simulink model "Synchrouns_Buck_Converter"  (R2022b)
settings: Solver=FixedStepAuto  StartTime=0.0  StopTime=inf  MaxStep=1e-5  RelTol=1e-3  EnableMultiTasking=on
libraries: spsSeriesRLCBranchLib x3, arduinolib x2, spsCurrentMeasurementLib x2, spsMosfetLib x2, spsVoltageMeasurementLib x2, spsDCVoltageSourceLib x1, spsFirstOrderFilterLib x1, dspstat3 x1, slpidlib x1, simulink x1, spspowerguiLib x1
settings Model: ExtModeTrigDuration=2  Creator=es-ahmedabdellatif20  LastModifiedBy=es-ahmedabdellatif20
settings OptimizationCC: EnhancedBackFolding=on  PassReuseOutputArgsAs=Individual arguments  ZeroExternalMemoryAtStartup=off  ZeroInternalMemoryAtStartup=off  MaxStackSize=64  OptimizeBlockOrder=speed  DifferentSizesBufferReuse=on  OptimizationCustomize=off  EfficientTunableParamExpr=on
settings DebuggingCC: ParameterTunabilityLossMsg=error
settings HardwareCC: ProdBitPerInt=16  ProdBitPerPointer=16  ProdBitPerSizeT=16  ProdBitPerPtrDiffT=16  ProdLargestAtomicFloat=None  ProdWordSize=8  ProdHWDeviceType=Atmel->AVR
settings SFSimCC: MATLABDynamicMemAlloc=off
settings RTWCC: Description=Embedded Coder  SystemTargetFile=ert.tlc  HardwareBoard=Arduino Uno  TLCOptions=-aInlineSetEventsForThisBaseRateFcn=TLC_FALSE -aSuppressMultiTaskScheduler=TLC_FALSE -aRateBasedStepFcn=1  TemplateMakefile=ert_default_tmf  Toolchain=Arduino AVR  BuildConfiguration=Faster Runs
settings CodeAppCC: ForceParamTrailComments=on  IgnoreCustomStorageClasses=off  OperatorAnnotations=on  SimulinkDataObjDesc=on  SFDataObjDesc=on  InsertBlockDesc=on
settings ERTTargetCC: SupportContinuousTime=on  SupportVariableSizeSignals=on  ExtModeTransport=3  ExtModeStaticAlloc=on  ExtModeAutomaticAllocSize=off  ExtModeStaticAllocSize=250  ExtModeMexFile=ext_xcp  ExtModeIntrfLevel=Level2 - Open

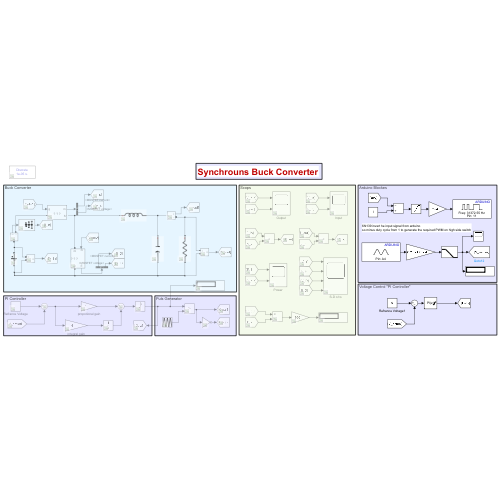
[thumbnail: Simulink's stored preview of the top-level diagram]
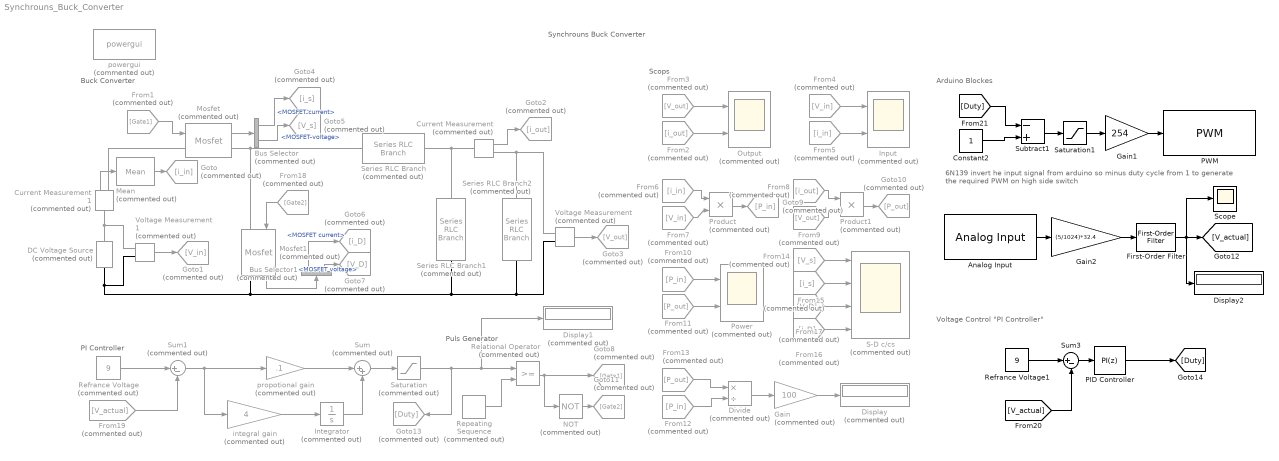
== system Synchrouns_Buck_Converter ==
  note: Voltage Control "PI Controller"
  note: 6N139 invert he input signal from arduino
      | so minus duty cycle from 1 to generate the required PWM on high side switch
  note: Arduino Blockes
  note: Scops
  note: Synchrouns Buck Converter
  note: Puls Generator
  note: PI Controller
  note: Buck Converter
  Analog Input : arduinolib/Analog Input  pinNumber=4  ReadResultsOnly=off  ConversionTriggerSource=Software  ExternalTriggerType=uint32( 0 )  OutputDataType=uint16  EnableConversionCompleteNotify=off  EnableOuputStatus=off  SampleTime=1e-3  blockPlatform=arduino
  Bus Selector : BusSelector  Commented=on  OutputSignals=MOSFET current,MOSFET voltage
  Bus Selector1 : BusSelector  Commented=on  OutputSignals=MOSFET current,MOSFET voltage
  Constant2 : Constant
  Current Measurement : spsCurrentMeasurementLib/Current Measurement  Commented=on  PhasorSimulation=off  OutputType=Complex  PSBequivalent=0
  Current Measurement1 : spsCurrentMeasurementLib/Current Measurement  Commented=on  PhasorSimulation=off  OutputType=Complex  PSBequivalent=0
  DC Voltage Source : spsDCVoltageSourceLib/DC Voltage Source  Commented=on  Amplitude=12  Measurements=Voltage
  Display : Display  Commented=on
  Display1 : Display  Commented=on
  Display2 : Display
  Divide : Product  Commented=on  Inputs=*/
  First-Order Filter : spsFirstOrderFilterLib/First-Order Filter  FilterType=Lowpass  Tc=1/250  Ts=1e-3  Initialize=off  Vac_Init=[0, 0, 60]  Vdc_Init=0  PlotResponse=off  FreqRange="[0,  200,  1]"
  From1 : From  Commented=on  GotoTag=Gate1
  From10 : From  Commented=on  GotoTag=P_in
  From11 : From  Commented=on  GotoTag=P_out
  From12 : From  Commented=on  GotoTag=P_in
  From13 : From  Commented=on  GotoTag=P_out
  From14 : From  Commented=on  GotoTag=V_s
  From15 : From  Commented=on  GotoTag=i_s
  From16 : From  Commented=on  GotoTag=i_D
  From17 : From  Commented=on  GotoTag=V_D
  From18 : From  Commented=on  GotoTag=Gate2
  From19 : From  Commented=on  GotoTag=V_actual
  From2 : From  Commented=on  GotoTag=i_out
  From3 : From  Commented=on  GotoTag=V_out
  From4 : From  Commented=on  GotoTag=V_in
  From5 : From  Commented=on  GotoTag=i_in
  From6 : From  Commented=on  GotoTag=i_in
  From7 : From  Commented=on  GotoTag=V_in
  From8 : From  Commented=on  GotoTag=i_out
  From9 : From  Commented=on  GotoTag=V_out
  Gain : Gain  Commented=on  Gain=100
  Gain1 : Gain  Gain=254
  Gain2 : Gain  Gain=(5/1024)*32.4
  Goto : Goto  Commented=on  GotoTag=i_in
  Goto1 : Goto  Commented=on  GotoTag=V_in
  Goto10 : Goto  Commented=on  GotoTag=P_out
  Goto11 : Goto  Commented=on  GotoTag=Gate2
  Goto13 : Goto  Commented=on  GotoTag=Duty
  Goto2 : Goto  Commented=on  GotoTag=i_out
  Goto3 : Goto  Commented=on  GotoTag=V_out
  Goto4 : Goto  Commented=on  GotoTag=i_s
  Goto5 : Goto  Commented=on  GotoTag=V_s
  Goto6 : Goto  Commented=on  GotoTag=i_D
  Goto7 : Goto  Commented=on  GotoTag=V_D
  Goto8 : Goto  Commented=on  GotoTag=Gate1
  Goto9 : Goto  Commented=on  GotoTag=P_in
  Input : Scope  Commented=on  NumInputPorts=2
  Integrator : Integrator  Commented=on
  Mean : dspstat3/Mean  Commented=on  run=on  InputProcessing=Columns as channels (frame based)  reset_popup=None  directionMode=Each column  dimension=1  roiEnable=off  roiType=Rectangles  roiPortion=Entire ROI  roiOutput=Individual statistics for each ROI  roiFlag=off  roundingMode=Floor  overflowMode=off  outputDataTypeStr=Inherit: Same as accumulator  outputMin=[]  outputMax=[]  outputLastDataTypeStr=Inherit: Same as accumulator
  Mosfet : spsMosfetLib/Mosfet  Commented=on  Ron=0.1  Lon=0  Rd=0.01  Vfd=0  IC=0  Rs=1e5  Cs=inf  Measurements=on
  Mosfet1 : spsMosfetLib/Mosfet  Commented=on  Ron=0.1  Lon=0  Rd=0.01  Vfd=0  IC=0  Rs=1e5  Cs=inf  Measurements=on
  NOT : Logic  Commented=on  Operator=NOT  IconShape=distinctive  AllPortsSameDT=off  OutDataTypeStr=boolean
  Output : Scope  Commented=on  NumInputPorts=2
  PID Controller : slpidlib/PID Controller  Controller=PI  Form=Parallel  TimeDomain=Discrete-time  UseExternalTs=off  SampleTime=1e-3  IntegratorMethod=Forward Euler  FilterMethod=Forward Euler  ControllerParametersSource=internal  P=.1  I=6  UseKiTs=off  D=0  N=100  UseFilter=on  TunerSelectOption=Transfer Function Based (PID Tuner App)  InitialConditionSource=internal  InitialConditionForIntegrator=0  InitialConditionForFilter=0  DifferentiatorICPrevScaledInput=0  ExternalReset=none  TrackingMode=off  Kt=1  LimitOutput=on  SatLimitsSource=internal  UpperSaturationLimit=1  LowerSaturationLimit=0  LinearizeAsGain=on  AntiWindupMode=clamping  Kb=1  LimitIntegrator=off  UpperIntegratorSaturationLimit=inf  LowerIntegratorSaturationLimit=-inf  POutMin=[]  POutMax=[]  IOutMin=[]  IOutMax=[]  DOutMin=[]  DOutMax=[]  NOutMin=[]  NOutMax=[]  SumOutMin=[]  SumOutMax=[]  SaturationOutMin=[]  SaturationOutMax=[]  PParamMin=[]  PParamMax=[]  IParamMin=[]  IParamMax=[]  DParamMin=[]  DParamMax=[]  NParamMin=[]  NParamMax=[]  KbParamMin=[]  KbParamMax=[]  KtParamMin=[]  KtParamMax=[]  KbOutMin=[]  KbOutMax=[]  KtOutMin=[]  KtOutMax=[]  IntegratorOutMin=[]  IntegratorOutMax=[]  FilterOutMin=[]  FilterOutMax=[]  SumI1OutMin=[]  SumI1OutMax=[]  SumI2OutMin=[]  SumI2OutMax=[]  SumI3OutMin=[]  SumI3OutMax=[]  SumI4OutMin=[]  SumI4OutMax=[]  SumDOutMin=[]  SumDOutMax=[]  DifferentiatorOutMin=[]  DifferentiatorOutMax=[]  FilterDiffOutCoefMin=[]  FilterDiffOutCoefMax=[]  ReciprocalOutMin=[]  ReciprocalOutMax=[]  SumDenOutMin=[]  SumDenOutMax=[]  SumNumOutMin=[]  SumNumOutMax=[]  DivideOutMin=[]  DivideOutMax=[]  UdiffTsProdOutMin=[]  UdiffTsProdOutMax=[]  NTsProdOutMin=[]  NTsProdOutMax=[]  UintegralTsProdOutMin=[]  UintegralTsProdOutMax=[]  UngainTsProdOutMin=[]  UngainTsProdOutMax=[]  ClampingZeroOutDataTypeStr=Inherit: Inherit via back propagation  ClampingZeroOutMin=[]  ClampingZeroOutMax=[]  FilterDenConstantOutDataTypeStr=Inherit: Inherit via back propagation  FilterDenConstantOutMin=[]  FilterDenConstantOutMax=[]  PCopyOutDataTypeStr=Inherit: Inherit via back propagation  PCopyOutMin=[]  PCopyOutMax=[]  NCopyOutDataTypeStr=Inherit: Inherit via back propagation  NCopyOutMin=[]  NCopyOutMax=[]  IntegratorContinuousStateAttributes=''  IntegratorStateMustResolveToSignalObject=off  IntegratorRTWStateStorageClass=Auto  FilterContinuousStateAttributes=''  FilterStateMustResolveToSignalObject=off  FilterRTWStateStorageClass=Auto  ParallelPVariant=InternalParameters  IdealPVariant=Disabled  IVariant=InternalParameters  DVariant=Disabled  IntegratorVariant=Discrete  SatVariant=Enabled  AWVariant=DiscClampingParallel  PCopyVariant=Disabled  TRVariant=Disabled  FdbkBlocksVariant=Forward  IdealPFdbkVariant=Disabled  SatFdbkVariant=Disabled  DerivativeFilterVariant=Disabled  NVariant=Disabled  NCopyVariant=Disabled_SignalSpec  FilterICVariant=Disabled  IntegratorICVariant=InternalICs  ExternalResetVariant=Disabled  TRSumVariant=Passthrough  SumFdbkVariant=Disabled  SumVariant=Sum_PI  TsampFilterVariant=InternalTs  TsampNgainVariant=Passthrough  TsampIntegralVariant=Passthrough  ExternalSaturationOutDataTypeStr=Inherit: Same as second input
  PWM : arduinolib/PWM  pinNumber=11  frequencyType=Specify  desiredFrequency=31372.55  achievableFrequency=31372.55
  Power : Scope  Commented=on  NumInputPorts=2
  Product : Product  Commented=on
  Product1 : Product  Commented=on
  Refrance Voltage : Constant  Commented=on  Value=9
  Refrance Voltage1 : Constant  Value=9
  Relational Operator : RelationalOperator  Commented=on  OutDataTypeStr=boolean  RndMeth=Simplest  InputSameDT=off
  Repeating Sequence : simulink/Sources/Repeating Sequence  Commented=on  rep_seq_t=[0 1/(31372.55*2) 1/31372.55]  rep_seq_y=[0 1 0]
  S-D c/cs : Scope  Commented=on  NumInputPorts=4
  Saturation : Saturate  Commented=on  UpperLimit=1  LowerLimit=0
  Saturation1 : Saturate  UpperLimit=1  LowerLimit=0
  Scope : Scope
  Series RLC Branch : spsSeriesRLCBranchLib/Series RLC Branch  Commented=on  LConnTagsString=__new0  RConnTagsString=__new0  BranchType=L  Resistance=1  Inductance=4e-3  SetiL0=off  InitialCurrent=0  Capacitance=1e-6  Setx0=off  InitialVoltage=0  Measurements=None
  Series RLC Branch1 : spsSeriesRLCBranchLib/Series RLC Branch  Commented=on  LConnTagsString=__new0  RConnTagsString=__new0  BranchType=C  Resistance=1  Inductance=1e-3  SetiL0=off  InitialCurrent=0  Capacitance=2200e-6  Setx0=off  InitialVoltage=0  Measurements=None
  Series RLC Branch2 : spsSeriesRLCBranchLib/Series RLC Branch  Commented=on  LConnTagsString=__new0  RConnTagsString=__new0  BranchType=R  Resistance=1  Inductance=1e-3  SetiL0=off  InitialCurrent=0  Capacitance=1e-6  Setx0=off  InitialVoltage=0  Measurements=None
  Subtract1 : Sum  Inputs=-+
  Sum : Sum  Commented=on  Inputs=|++
  Sum1 : Sum  Commented=on  Inputs=|+-
  Sum3 : Sum  Inputs=|+-
  Voltage Measurement : spsVoltageMeasurementLib/Voltage Measurement  Commented=on  PhasorSimulation=off  OutputType=Complex  PSBequivalent=0
  Voltage Measurement1 : spsVoltageMeasurementLib/Voltage Measurement  Commented=on  PhasorSimulation=off  OutputType=Complex  PSBequivalent=0
  integral gain : Gain  Commented=on  Gain=4
  powergui : spspowerguiLib/powergui  Priority=1  Commented=on  SimulationMode=Discrete  SampleTime=1e-5  frequency=60  Iterations=50  frequencyindice=0  Pbase=100e6  ErrMax=1e-4  UnitsV=kV  UnitsW=MW  buscounter=0  FunctionMessages=off  echomessages=off  EnableUseOfTLC=off  CurrentSourceSwitches=off  DisableSnubberDevices=off  DisableRonSwitches=off  DisableVfSwitches=off  DisplayEquations=off  AutomaticDiscreteSolvers=off  SolverType=Tustin/Backward Euler (TBE)  Interpol=off  ExternalGateDelay=off  methode=off  Ts=100  x0status=blocks  SPID=on  SwTol=0  HookPort=off  NonlinearTolerance=1e-4  nMaxIteration=100  ContinueOnMaxIteration=off  RestoreLinks=warning  ResistiveCurrentMeasurement=off  Frange=[0:2:500]  Ylog=off  Xlog=on  ShowGrid=off  save=off  variable=ZData  structure=0  ZoomFFT=off  StartTime=0.0  cycles=1  DisplayStyle=1  fundamental=60  FreqAxis=off  MaxFrequency=1000  frequencyindicesteady=1  RmsSteady=1  display=off
  propotional gain : Gain  Commented=on  Gain=.1
  wires:
  Voltage Measurement1/1 -> Goto1/1
  Current Measurement/1 -> Goto2/1
  Voltage Measurement/1 -> Goto3/1
  Mosfet/1 -> Bus Selector/1
  Mosfet1/1 -> Bus Selector1/1
  Bus Selector/1 -> Goto4/1  "<MOSFET current>"
  Bus Selector/2 -> Goto5/1  "<MOSFET voltage>"
  Bus Selector1/1 -> Goto6/1  "<MOSFET current>"
  integral gain/1 -> Integrator/1
  Integrator/1 -> Sum/2
  propotional gain/1 -> Sum/1
  Sum/1 -> Saturation/1
  Relational Operator/1 -> Goto8/1, NOT/1
  Refrance Voltage/1 -> Sum1/1
  Sum1/1 -> integral gain/1, propotional gain/1
  From1/1 -> Mosfet/1
  Bus Selector1/2 -> Goto7/1  "<MOSFET voltage>"
  Repeating Sequence/1 -> Relational Operator/2
  From3/1 -> Output/1
  From2/1 -> Output/2
  From5/1 -> Input/2
  From4/1 -> Input/1
  From6/1 -> Product/1
  From7/1 -> Product/2
  From9/1 -> Product1/2
  From8/1 -> Product1/1
  Product/1 -> Goto9/1
  Product1/1 -> Goto10/1
  From10/1 -> Power/1
  From11/1 -> Power/2
  From13/1 -> Divide/1
  From12/1 -> Divide/2
  Divide/1 -> Gain/1
  Gain/1 -> Display/1
  From14/1 -> S-D c/cs/1
  From15/1 -> S-D c/cs/2
  From17/1 -> S-D c/cs/3
  From16/1 -> S-D c/cs/4
  Current Measurement1/1 -> Mean/1
  Mean/1 -> Goto/1
  NOT/1 -> Goto11/1
  From18/1 -> Mosfet1/1
  Gain1/1 -> PWM/1
  Saturation1/1 -> Gain1/1
  Saturation/1 -> Goto13/1, Display1/1, Relational Operator/1
  Analog Input/1 -> Gain2/1
  Constant2/1 -> Subtract1/2
  Subtract1/1 -> Saturation1/1
  From19/1 -> Sum1/2
  [V_actual] -> Sum3/2
  Refrance Voltage1/1 -> Sum3/1
  Sum3/1 -> PID Controller/1
  PID Controller/1 -> [Duty]
  [Duty] -> Subtract1/1
  Gain2/1 -> First-Order Filter/1
  First-Order Filter/1 -> Display2/1, [V_actual], Scope/1
  connections:
  Mosfet/LConn1 -- Current Measurement1/RConn1
  Series RLC Branch/LConn1 -- Mosfet1/LConn1 -- Mosfet/RConn1
  DC Voltage Source/LConn1 -- Series RLC Branch2/RConn1 -- Voltage Measurement/LConn2 -- Series RLC Branch1/RConn1 -- Mosfet1/RConn1 -- Voltage Measurement1/LConn2
  Series RLC Branch1/LConn1 -- Current Measurement/LConn1 -- Series RLC Branch/RConn1
  Voltage Measurement/LConn1 -- Series RLC Branch2/LConn1 -- Current Measurement/RConn1
  Voltage Measurement1/LConn1 -- Current Measurement1/LConn1 -- DC Voltage Source/RConn1
